simulink model "knee_jerk_v1"  (R2022a)
settings: Solver=VariableStepAuto  StartTime=0.0  StopTime=60  RelTol=1e-3
undefined symbols (not defined in the file): beta, K, L, m, M
settings Model: Creator=kabil  LastModifiedBy=kabil

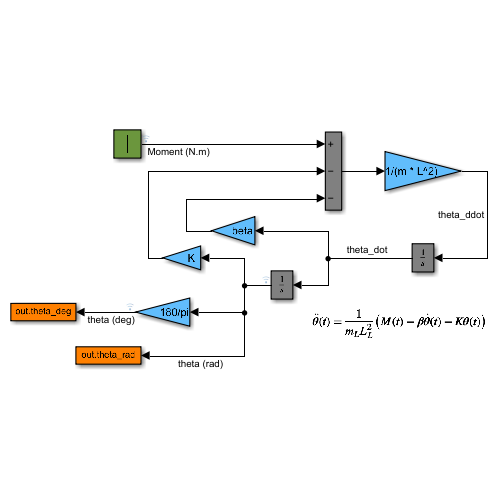
[thumbnail: Simulink's stored preview of the top-level diagram]
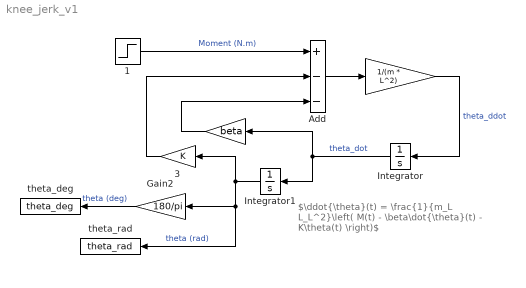
== system knee_jerk_v1 ==
  note: $\ddot{\theta}(t) = \frac{1}{m_L L_L^2}\left( M(t) - \beta\dot{\theta}(t) - K\theta(t) \right)$
  "  " : Gain  Gain=1/(m * L^2)
  "   " : Gain  Gain=beta
  1 : Step  After=M  SampleTime=0
  3 : Gain  Gain=K
  Add : Sum  Inputs=+--
  Gain2 : Gain  Gain=180/pi
  Integrator : Integrator
  Integrator1 : Integrator
  theta_deg : ToWorkspace  VariableName=theta_deg  SampleTime=-1
  theta_rad : ToWorkspace  VariableName=theta_rad  SampleTime=-1
  wires:
  Integrator/1 -> Integrator1/1, "   "/1  "theta_dot"
  3/1 -> Add/2
  1/1 -> Add/1  "Moment (N.m)"
  Integrator1/1 -> theta_rad/1, Gain2/1, 3/1  "theta (rad)"
  Add/1 -> "  "/1
  "   "/1 -> Add/3
  "  "/1 -> Integrator/1  "theta_ddot"
  Gain2/1 -> theta_deg/1  "theta (deg)"
